simulink model "torque_tau_r"  (R2022b)
settings: Solver=VariableStepAuto  StartTime=0.0  StopTime=10.0  RelTol=1e-3
model workspace (MAT data in the model file):
  J_motor = Simulink.Parameter
  J_motor.Value = 2e-05
  J_motor.DataType = 'auto'
  J_motor.Complexity = 'real'
  J_motor.Dimensions = [1 1]
  J_robot = Simulink.Parameter
  J_robot.Value = 5e-05
  J_robot.DataType = 'auto'
  J_robot.Complexity = 'real'
  J_robot.Dimensions = [1 1]
  K_motor = Simulink.Parameter
  K_motor.Value = 0.25
  K_motor.DataType = 'auto'
  K_motor.Complexity = 'real'
  K_motor.Dimensions = [1 1]
  K_robot = Simulink.Parameter
  K_robot.Value = 0.2
  K_robot.DataType = 'auto'
  K_robot.Complexity = 'real'
  K_robot.Dimensions = [1 1]
libraries: slpidlib x1
settings Model: Creator=saayu  LastModifiedBy=saayu

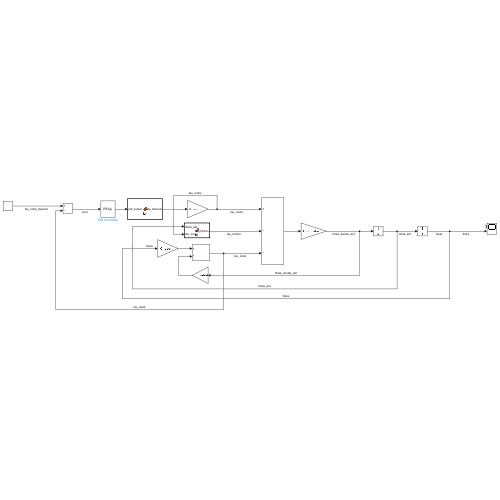
[thumbnail: Simulink's stored preview of the top-level diagram]
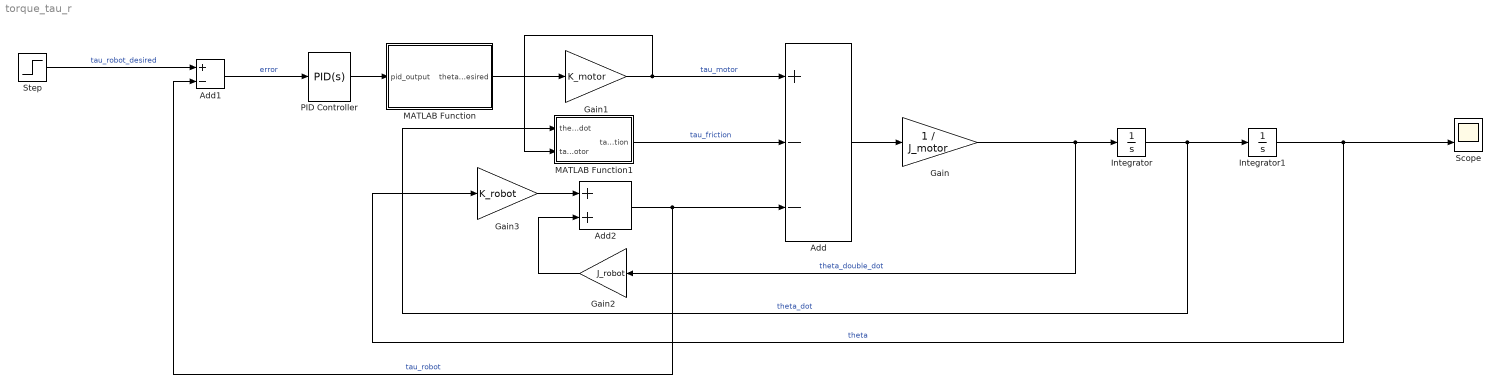
== system torque_tau_r ==
  Add : Sum  Inputs=+--
  Add1 : Sum  Inputs=+-
  Add2 : Sum
  Gain : Gain  Gain=1 / J_motor
  Gain1 : Gain  Gain=K_motor
  Gain2 : Gain  Gain=J_robot
  Gain3 : Gain  Gain=K_robot
  Integrator : Integrator
  Integrator1 : Integrator
  MATLAB Function : MATLAB Function  TreatAsAtomicUnit=on
  MATLAB Function1 : MATLAB Function  TreatAsAtomicUnit=on
  PID Controller : slpidlib/PID Controller  Controller=PID  Form=Parallel  TimeDomain=Continuous-time  UseExternalTs=off  SampleTime=-1  IntegratorMethod=Forward Euler  FilterMethod=Forward Euler  ControllerParametersSource=internal  P=10  I=10  UseKiTs=off  D=10  N=100  UseFilter=on  TunerSelectOption=Transfer Function Based (PID Tuner App)  InitialConditionSource=internal  InitialConditionForIntegrator=0  InitialConditionForFilter=0  DifferentiatorICPrevScaledInput=0  ExternalReset=none  TrackingMode=off  Kt=1  LimitOutput=off  SatLimitsSource=internal  UpperSaturationLimit=inf  LowerSaturationLimit=-inf  LinearizeAsGain=on  AntiWindupMode=none  Kb=1  LimitIntegrator=off  UpperIntegratorSaturationLimit=inf  LowerIntegratorSaturationLimit=-inf  POutMin=[]  POutMax=[]  IOutMin=[]  IOutMax=[]  DOutMin=[]  DOutMax=[]  NOutMin=[]  NOutMax=[]  SumOutMin=[]  SumOutMax=[]  SaturationOutMin=[]  SaturationOutMax=[]  PParamMin=[]  PParamMax=[]  IParamMin=[]  IParamMax=[]  DParamMin=[]  DParamMax=[]  NParamMin=[]  NParamMax=[]  KbParamMin=[]  KbParamMax=[]  KtParamMin=[]  KtParamMax=[]  KbOutMin=[]  KbOutMax=[]  KtOutMin=[]  KtOutMax=[]  IntegratorOutMin=[]  IntegratorOutMax=[]  FilterOutMin=[]  FilterOutMax=[]  SumI1OutMin=[]  SumI1OutMax=[]  SumI2OutMin=[]  SumI2OutMax=[]  SumI3OutMin=[]  SumI3OutMax=[]  SumI4OutMin=[]  SumI4OutMax=[]  SumDOutMin=[]  SumDOutMax=[]  DifferentiatorOutMin=[]  DifferentiatorOutMax=[]  FilterDiffOutCoefMin=[]  FilterDiffOutCoefMax=[]  ReciprocalOutMin=[]  ReciprocalOutMax=[]  SumDenOutMin=[]  SumDenOutMax=[]  SumNumOutMin=[]  SumNumOutMax=[]  DivideOutMin=[]  DivideOutMax=[]  UdiffTsProdOutMin=[]  UdiffTsProdOutMax=[]  NTsProdOutMin=[]  NTsProdOutMax=[]  UintegralTsProdOutMin=[]  UintegralTsProdOutMax=[]  UngainTsProdOutMin=[]  UngainTsProdOutMax=[]  ClampingZeroOutDataTypeStr=Inherit: Inherit via back propagation  ClampingZeroOutMin=[]  ClampingZeroOutMax=[]  FilterDenConstantOutDataTypeStr=Inherit: Inherit via back propagation  FilterDenConstantOutMin=[]  FilterDenConstantOutMax=[]  PCopyOutDataTypeStr=Inherit: Inherit via back propagation  PCopyOutMin=[]  PCopyOutMax=[]  NCopyOutDataTypeStr=Inherit: Inherit via back propagation  NCopyOutMin=[]  NCopyOutMax=[]  IntegratorContinuousStateAttributes=''  IntegratorStateMustResolveToSignalObject=off  IntegratorRTWStateStorageClass=Auto  FilterContinuousStateAttributes=''  FilterStateMustResolveToSignalObject=off  FilterRTWStateStorageClass=Auto  ParallelPVariant=InternalParameters  IdealPVariant=Disabled  IVariant=InternalParameters  DVariant=InternalParameters  IntegratorVariant=Continuous  SatVariant=Disabled  AWVariant=Passthrough  PCopyVariant=Disabled  TRVariant=Disabled  FdbkBlocksVariant=Forward  IdealPFdbkVariant=Disabled  SatFdbkVariant=Disabled  DerivativeFilterVariant=ContFilter  NVariant=InternalParameters  NCopyVariant=Disabled  FilterICVariant=InternalICsFilter  IntegratorICVariant=InternalICs  ExternalResetVariant=Disabled  TRSumVariant=Passthrough  SumFdbkVariant=Disabled  SumVariant=Sum_PID  TsampFilterVariant=InternalTs  TsampNgainVariant=Passthrough  TsampIntegralVariant=Passthrough  ExternalSaturationOutDataTypeStr=Inherit: Same as second input
  Scope : Scope  NumInputPorts=2
  Step : Step  SampleTime=0
  wires:
  Step/1 -> Add1/1  "tau_robot_desired"
  Integrator1/1 -> Scope/2, Gain3/1  "theta"
  Gain1/1 -> MATLAB Function1/2(tau_motor), Add/1  "tau_motor"
  Gain2/1 -> Add2/2
  Gain3/1 -> Add2/1
  Add1/1 -> PID Controller/1  "error"
  Add2/1 -> Add1/2, Add/3  "tau_robot"
  Gain/1 -> Gain2/1, Integrator/1  "theta_double_dot"
  Integrator/1 -> MATLAB Function1/1(theta_dot), Integrator1/1  "theta_dot"
  MATLAB Function1/1(tau_friction) -> Add/2  "tau_friction"
  Add/1 -> Gain/1
  PID Controller/1 -> MATLAB Function/1(pid_output)
  MATLAB Function/1(theta_desired) -> Gain1/1

== matlab function torque_tau_r/MATLAB Function ==
  data: pid_output input; theta_desired output
function theta_desired = fcn(pid_output)

% function to convert the pid output and feed it to the motor
theta_desired = pid_output;

== matlab function torque_tau_r/MATLAB Function1 ==
  data: theta_dot input; tau_friction output; tau_motor input
function tau_friction = fcn(theta_dot, tau_motor)

if theta_dot == 0
    tau_friction = tau_motor;
elseif theta_dot > 0
    tau_friction = 0.05;
else
    tau_friction = - 0.05;
end
